simulink library "NCS_Library"  (R2019a)
settings: Solver=VariableStepAuto  StartTime=0.0  StopTime=10.0  RelTol=1e-3
values from neighbouring files (symbols this model uses):
  A = 10    [Parameter.m]
  band = 100000000    [Parameter.m]
  BER = 0    [Parameter.m]
  c = 5000000    [Parameter.m]
  c1 = 4.33    [Parameter.m]
  c2 = 3.16    [Parameter.m]
  CAN2EthernetDelay = 0.000    (= 0)    [Parameter.m]
  cR = 1.5*10^-3    (= 0.0015)    [Parameter.m]
  cw = (cwE * 2 + cwM * (nW_ges-2))/nW_ges    (= 0.1475)    [Parameter.m]
  cwE = 0.35    [Parameter.m]
  cwM = 0.08    [Parameter.m]
  Cycle_Controller = 0    [Parameter.m]
  CyclePLC = 24/1000    (= 0.024)    [Parameter.m]
  d = 800000    [Parameter.m]
  Dr = 0.92    [Parameter.m]
  Ethernet2CANDelay = 0.005    [Parameter.m]
  F_konst = 70892    [Parameter.m]
  FA = 100000    [Parameter.m]
  FB_WB_max = 10000    [Parameter.m]
  FBel_an = iG*nG*F_KZmax*nBan*R_mR/(Dr/2)    (= 28197.4297239)    [Parameter.m]
  FBel_frei = iG*nG*F_KZmax*nBfrei*R_mW/(Dr/2)    (= 29270.6882948)    [Parameter.m]
  Fmaxdyn = 300000    [Parameter.m]
  g = 9.81    [Parameter.m]
  i = 0    [Parameter.m]
  J = 1/2*mA*(Dr/2)^2    (= 158.7)    [Parameter.m]
  k1 = 0.095    [Parameter.m]
  k2 = 9.26/3.6    (= 2.57222222222)    [Parameter.m]
  k3 = 4.63/3.6    (= 1.28611111111)    [Parameter.m]
  mges = 58000    [Parameter.m]
  mu = [mu1 mu2]    [Parameter.m]
  muBel1 = 0.42    [Parameter.m]
  muBel2 = 0.36    [Parameter.m]
  n = 0.001    [Parameter.m]
  n_Mg = 4    [Parameter.m]
  n_WB = 4    [Parameter.m]
  nA = 4    [Parameter.m]
  nBan = 2    [Parameter.m]
  nBfrei = 3    [Parameter.m]
  nM = 4    [Parameter.m]
  nW_an = 4    [Parameter.m]
  P_max = 8200000    [Parameter.m]
  Q = 10    [Parameter.m]
  r_reib = 600    [Parameter.m]
  rho = 1.08    [Parameter.m]
  rhoL = 1.225    [Parameter.m]
  Size = 8    [Parameter.m]
  slip = [s1 s2]    [Parameter.m]
  tol = 0.05    [Parameter.m]
  v00 = 100/3.6    (= 27.7777777778)    [Parameter.m]
  v_grenz = 60/3.6    (= 16.6666666667)    [Parameter.m]
  v_opt = 75/3.6    (= 20.8333333333)    [Parameter.m]
  W_opt = 0.5    [Parameter.m]
  WB = 1    [Parameter.m]
  y_opt = sqrt(W_opt)/((1+sqrt(W_opt))^2+W_opt)    [Parameter.m]
undefined symbols (not defined in the file or in its folder): BUSCapacity, CableLength, controlGate, D_dyn, D_mg, EnableBurst, EnableToF, entity, Entity_out, Gate, Gate_4, Gate_5, Gate_ACK, Gate_copy, Gate_RX, getData, gettime, I_dyn, I_mg, m, magnitude, P_dyn, P_mg, ReadAttributes, readdata, ReadData, ReadSize, sigbuilder_block, Timeout, ToB, ToF, v0, v_d, v_soll
libraries: simulink x176, $bdroot x102
(part 10 of 12)

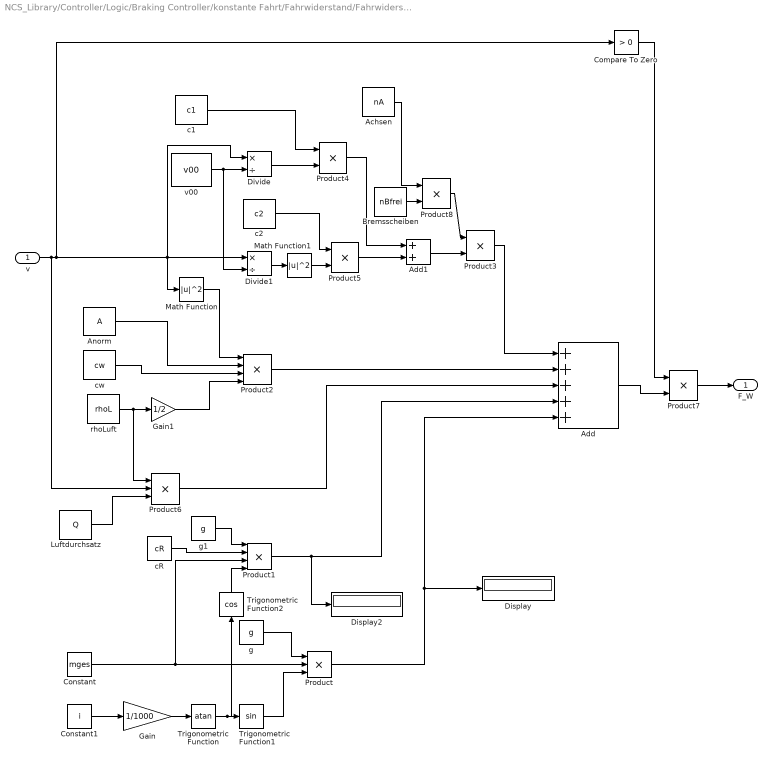
== system NCS_Library/Controller/Logic/Braking Controller/konstante Fahrt/Fahrwiderstand/Fahrwiderstand_freiWagen ==
  v : Inport
  Achsen : Constant  Value=nA
  Add : Sum  Inputs=+++++
  Add1 : Sum
  Anorm : Constant  Value=A
  Bremsscheiben : Constant  Value=nBfrei
  Compare To Zero : simulink/Logic and Bit Operations/Compare To Zero  relop=>  OutDataTypeStr=boolean
  Constant : Constant  Value=mges
  Constant1 : Constant  Value=i
  Display : Display
  Display2 : Display
  Divide : Product  Inputs=*/
  Divide1 : Product  Inputs=*/
  Gain : Gain  Gain=1/1000
  Gain1 : Gain  Gain=1/2
  Luftdurchsatz : Constant  Value=Q
  Math Function : Math  Operator=magnitude^2  SaturateOnIntegerOverflow=on
  Math Function1 : Math  Operator=magnitude^2  SaturateOnIntegerOverflow=on
  Product : Product  Inputs=3
  Product1 : Product  Inputs=4
  Product2 : Product  Inputs=4
  Product{3..5,7..8} (5 alike) : Product
  Product6 : Product  Inputs=3
  Trigonometric Function : Trigonometry  Operator=atan
  Trigonometric Function1 : Trigonometry
  Trigonometric Function2 : Trigonometry  Operator=cos
  c1 : Constant  Value=c1
  c2 : Constant  Value=c2
  cR : Constant  Value=cR
  cw : Constant  Value=cw
  g : Constant  Value=g
  g1 : Constant  Value=g
  rhoLuft : Constant  Value=rhoL
  v00 : Constant  Value=v00
  F_W : Outport
  wires:
  Trigonometric Function2/1 -> Product1/4
  Constant/1 -> Product1/3, Product/2
  cR/1 -> Product1/2
  g1/1 -> Product1/1
  Gain/1 -> Trigonometric Function/1
  Trigonometric Function/1 -> Trigonometric Function1/1, Trigonometric Function2/1
  Constant1/1 -> Gain/1
  Bremsscheiben/1 -> Product8/2
  Product8/1 -> Product3/1
  Compare To Zero/1 -> Product7/1
  Product7/1 -> F_W/1
  Math Function1/1 -> Product5/2
  Product6/1 -> Add/3
  Luftdurchsatz/1 -> Product6/3
  c2/1 -> Product5/1
  Math Function/1 -> Product2/1
  Divide1/1 -> Math Function1/1
  Product5/1 -> Add1/2
  Product4/1 -> Add1/1
  Divide/1 -> Product4/2
  v00/1 -> Divide/2, Divide1/2
  c1/1 -> Product4/1
  Add1/1 -> Product3/2
  Product3/1 -> Add/1
  Achsen/1 -> Product8/1
  Product2/1 -> Add/2
  Gain1/1 -> Product2/4
  cw/1 -> Product2/3
  Anorm/1 -> Product2/2
  v/1 -> Math Function/1, Divide/1, Divide1/1, Compare To Zero/1, Product6/2
  rhoLuft/1 -> Gain1/1, Product6/1
  Product1/1 -> Add/4, Display2/1
  Add/1 -> Product7/2
  Product/1 -> Add/5, Display/1
  Trigonometric Function1/1 -> Product/3
  g/1 -> Product/1

== system NCS_Library/Controller/Logic/Braking Controller/konstante Fahrt/WB Bremse pro Wagen/Subsystem ==
  v : Inport
  Add : Sum
  Add1 : Sum
  Berechnung W : Subsystem
  Compare To Zero : simulink/Logic and Bit Operations/Compare To Zero  relop=>=  OutDataTypeStr=boolean
  Constant : Constant
  Display : Display
  Divide : Product  Inputs=*/
  Math Function : Math  Operator=magnitude^2  SaturateOnIntegerOverflow=on
  Product : Product
  Scope : Scope
  Sqrt : Sqrt  SaturateOnIntegerOverflow=on
  y : Outport
  wires:
  Compare To Zero/1 -> Product/1
  Berechnung W/1(W) -> Product/2, Compare To Zero/1
  Add1/1 -> Divide/2
  Divide/1 -> Scope/1, y/1
  Math Function/1 -> Add1/1
  Add/1 -> Math Function/1
  Constant/1 -> Add/2
  Sqrt/1 -> Divide/1, Add/1
  Product/1 -> Sqrt/1, Add1/2, Display/1
  v/1 -> Berechnung W/1(v)

== system NCS_Library/Network/CAN/Logik/Fast_to_Slow/Measurement/Enabled Subsystem3 ==
  time_arrived : Inport
  time_sent : Inport  Port=2
  Enable : EnablePort
  Add : Sum  Inputs=+-
  delay : Outport
  wires:
  Add/1 -> delay/1
  time_sent/1 -> Add/2
  time_arrived/1 -> Add/1

== system NCS_Library/Network/CAN/Logik/Fast_to_Slow/Measurement/Simulink Function7 ==
  getData : TriggerPort  TriggerType=function-call  IsSimulinkFunction=on  FunctionName=getData  FunctionVisibility=scoped  VariantControl=Variant
  u1 : ArgIn  DisableCoverage=on  ArgumentName=time
  time : Outport  InitialOutput=-1
  wires:
  u1/1 -> time/1

== system NCS_Library/Network/CAN/Logik/Fast_to_Slow/Slow Takt/Simulink Function3 ==
  Gate_5 : TriggerPort  TriggerType=function-call  IsSimulinkFunction=on  FunctionName=Gate_5  FunctionVisibility=scoped  VariantControl=Variant
  Message Send : MessageSend  OutputPortMessageModes=m
      settings: InputPortMap=u1
  u : ArgIn  DisableCoverage=on  ArgumentName=u
  ctrl : Outport  InitialOutput=0
  wires:
  Message Send/1 -> ctrl/1
  u/1 -> Message Send/1

== system NCS_Library/Network/CAN/Logik/Fast_to_Slow/Wait Takt/Simulink Function3 ==
  Gate_4 : TriggerPort  TriggerType=function-call  IsSimulinkFunction=on  FunctionName=Gate_4  FunctionVisibility=scoped  VariantControl=Variant
  Message Send : MessageSend  OutputPortMessageModes=m
      settings: InputPortMap=u1
  u : ArgIn  DisableCoverage=on  ArgumentName=u
  ctrl : Outport  InitialOutput=0
  wires:
  u/1 -> Message Send/1
  Message Send/1 -> ctrl/1

== system NCS_Library/Network/CAN/Logik/Slow_to_Fast/Copy Takt/Simulink Function3 ==
  Gate_copy : TriggerPort  TriggerType=function-call  IsSimulinkFunction=on  FunctionName=Gate_copy  FunctionVisibility=scoped  VariantControl=Variant
  Message Send : MessageSend  OutputPortMessageModes=m
      settings: InputPortMap=u1
  u : ArgIn  DisableCoverage=on  ArgumentName=u
  ctrl : Outport  InitialOutput=0
  wires:
  u/1 -> Message Send/1
  Message Send/1 -> ctrl/1

== system NCS_Library/Network/CAN/Logik/Slow_to_Fast/Fast Takt/Simulink Function3 ==
  Gate : TriggerPort  TriggerType=function-call  IsSimulinkFunction=on  FunctionName=Gate  FunctionVisibility=scoped  VariantControl=Variant
  Message Send : MessageSend  OutputPortMessageModes=m
      settings: InputPortMap=u1
  u : ArgIn  DisableCoverage=on  ArgumentName=u
  ctrl : Outport  InitialOutput=0
  wires:
  u/1 -> Message Send/1
  Message Send/1 -> ctrl/1

== system NCS_Library/Network/CAN/Logik/Slow_to_Fast/Logic Takt/Simulink Function3 ==
  Gate : TriggerPort  TriggerType=function-call  IsSimulinkFunction=on  FunctionName=Gate  FunctionVisibility=scoped  VariantControl=Variant
  Message Send : MessageSend  OutputPortMessageModes=m
      settings: InputPortMap=u1
  u : ArgIn  DisableCoverage=on  ArgumentName=u
  ctrl : Outport  InitialOutput=0
  wires:
  Message Send/1 -> ctrl/1
  u/1 -> Message Send/1

== system NCS_Library/Network/CAN/Logik/Slow_to_Fast/Measurement/Enabled Subsystem ==
  time_arrived : Inport
  time : Inport  Port=2
  Enable : EnablePort
  Add : Sum  Inputs=+-
  delay : Outport
  wires:
  time_arrived/1 -> Add/1
  time/1 -> Add/2
  Add/1 -> delay/1

== system NCS_Library/Network/CAN/Logik/Slow_to_Fast/Measurement/Fast Takt ==
  In : Inport
  Entity Takt : EntityGenerator  OutputPortMessageModes=m  TimeSource=Signal port  Period=7  AttributeName=entity  EntityTypeName=gate  EntityPriority=10  DataInitialValue=1
      settings: InputPortMap=u1
  Entity Terminator13 : EntityTerminator  InputPortMessageModes=m
  Gate : EntityGate  InputPortMessageModes=m,m  OutputPortMessageModes=m
  Offset [s] : Constant  Value=Offset
  Server : EntityServer  InputPortMessageModes=m  OutputPortMessageModes=m  Capacity=1  ServiceTimeValue=0  EntryAction=Gate(0);
  Server Offset : EntityServer  InputPortMessageModes=n,m  OutputPortMessageModes=m  Capacity=inf  ServiceTimeSource=Signal port  ServiceTimeValue=5
      settings: InputPortMap=u0,u2
  Server Takt : EntityServer  InputPortMessageModes=m  OutputPortMessageModes=m  Capacity=1  ServiceTimeValue=0.001  ServiceTimeAttributeName=CommDelay  EntryAction=Gate(1);  ExitAction=Gate(0);  SortingAttributeName=ID
  Simulink Function3 : Subsystem  TreatAsAtomicUnit=on
  Takt_fast [s] : Constant  Value=Takt_fast
  Out : Outport
  wires:
  Offset [s]/1 -> Server Offset/1
  Takt_fast [s]/1 -> Entity Takt/1
  Server Takt/1 -> Entity Terminator13/1
  Server Offset/1 -> Server Takt/1
  Entity Takt/1 -> Server Offset/2
  Simulink Function3/1(ctrl) -> Gate/1
  In/1 -> Gate/2
  Gate/1 -> Server/1
  Server/1 -> Out/1

== system NCS_Library/Network/CAN/Logik/Slow_to_Fast/Measurement/Simulink Function6 ==
  getData : TriggerPort  TriggerType=function-call  IsSimulinkFunction=on  FunctionName=getData  FunctionVisibility=scoped  VariantControl=Variant
  u : ArgIn  DisableCoverage=on  ArgumentName=time
  time : Outport  InitialOutput=-1
  wires:
  u/1 -> time/1

== system NCS_Library/Network/ETB/Burst Device/Protocl Stack/TRDP PD/Enabled Subsystem1 ==
  msgType : Inport
  ReplyAddress : Inport  Port=2
  Enable : EnablePort
  MATLAB Function : MATLAB Function  TreatAsAtomicUnit=on
  msgTypeReply : Outport  OutputWhenDisabled=reset  InitialOutput=0
  DestinationReply : Outport  Port=2
  wires:
  MATLAB Function/1(msgTypeReply) -> msgTypeReply/1
  ReplyAddress/1 -> DestinationReply/1
  msgType/1 -> MATLAB Function/1(msgType)

== system NCS_Library/Network/ETB/Burst Device/Protocl Stack/TRDP PD/Simulink Function ==
  msgType : Inport
  Destination : Inport  Port=2
  Source : Inport  Port=3
  UDP : Inport  Port=4
  ReplyAddress : Inport  Port=5
  f : TriggerPort  TriggerType=function-call  IsSimulinkFunction=on  FunctionName=SetAttributes  FunctionVisibility=scoped  VariantControl=(inherit)
  Constant : Constant  OutDataTypeStr=uint8
  Display : Display
  MATLAB Function : MATLAB Function  TreatAsAtomicUnit=on
  SSC : ArgIn  DisableCoverage=on  OutDataTypeStr=uint32  ArgumentName=SSC
  SSC1 : ArgIn  DisableCoverage=on  Port=2  PortDimensions=[3 20]  ArgumentName=Data
  y : ArgOut  DisableCoverage=on  OutDataTypeStr=uint32  ArgumentName=SEQ
  y1 : ArgOut  DisableCoverage=on  Port=2  OutDataTypeStr=uint8  ArgumentName=msgType
  y2 : ArgOut  DisableCoverage=on  Port=3  OutDataTypeStr=uint16  PortDimensions=[1 4]  ArgumentName=Destination
  y3 : ArgOut  DisableCoverage=on  Port=4  OutDataTypeStr=uint16  PortDimensions=[1 4]  ArgumentName=Source
  y5 : ArgOut  DisableCoverage=on  Port=5  OutDataTypeStr=uint8  ArgumentName=CheckBit
  y4 : ArgOut  DisableCoverage=on  Port=6  PortDimensions=[3 20]  ArgumentName=Data
  y6 : ArgOut  DisableCoverage=on  Port=7  OutDataTypeStr=uint16  ArgumentName=UDP
  y7 : ArgOut  DisableCoverage=on  Port=8  OutDataTypeStr=uint16  PortDimensions=[ 1 4 ]  ArgumentName=ReplyAddress
  wires:
  ReplyAddress/1 -> y7/1
  UDP/1 -> y6/1
  MATLAB Function/1(Data_edited) -> y4/1
  SSC1/1 -> MATLAB Function/1(Data)
  Constant/1 -> y5/1
  SSC/1 -> y/1
  Source/1 -> y3/1
  Destination/1 -> y2/1, Display/1
  msgType/1 -> y1/1, MATLAB Function/2(msgType)

== system NCS_Library/Network/ETB/Burst Device/Protocl Stack/TRDP PD/Simulink Function1 ==
  ReadData : TriggerPort  TriggerType=function-call  IsSimulinkFunction=on  FunctionName=ReadData  FunctionVisibility=scoped  VariantControl=(inherit)
  MATLAB Function : MATLAB Function  TreatAsAtomicUnit=on
  MATLAB Function2 : MATLAB Function  TreatAsAtomicUnit=on
  SourceAddress : ArgIn  DisableCoverage=on  OutDataTypeStr=uint8  ArgumentName=msgType
  SourceAddress1 : ArgIn  DisableCoverage=on  Port=2  OutDataTypeStr=uint16  PortDimensions=[1 4]  ArgumentName=Reply
  SourceAddress2 : ArgIn  DisableCoverage=on  Port=3  OutDataTypeStr=uint16  PortDimensions=[1 4]  ArgumentName=Source
  msgType : Outport  OutDataTypeStr=uint8  OutputWhenDisabled=reset  InitialOutput=0
  ReplyAddress : Outport  Port=2  OutDataTypeStr=uint16
  wires:
  MATLAB Function2/1(DestinationPull) -> ReplyAddress/1
  SourceAddress/1 -> MATLAB Function2/1(msgType), msgType/1
  MATLAB Function/1(Address) -> MATLAB Function2/2(ReplyAddress)
  SourceAddress2/1 -> MATLAB Function/2(Source)
  SourceAddress1/1 -> MATLAB Function/1(Reply)

== system NCS_Library/Network/ETB/OSI Layers/MAC Controller/CSMA//CD/Discrete Event Subsystem (Carrier Sensing)1 ==
  l_status : Inport
  Compare To Zero1 : simulink/Logic and Bit Operations/Compare To Zero  relop=>  OutDataTypeStr=boolean
  Constant1 : Constant
  Sum1 : Sum  Inputs=|+-
  l_ready : Outport  InitialOutput=1
  wires:
  Compare To Zero1/1 -> l_ready/1
  Sum1/1 -> Compare To Zero1/1
  l_status/1 -> Sum1/2
  Constant1/1 -> Sum1/1

== system NCS_Library/Network/ETB/OSI Layers/SDTv2/Safety Measures/Latency Monitoring ==
  Timestamp : Inport
  T_rx_safe : Inport  Port=2
  Enable : EnablePort
  Add1 : Sum  Inputs=+--+
  Clock : Clock
  Compare To Zero1 : simulink/Logic and Bit Operations/Compare To Zero  relop=>=  OutDataTypeStr=uint8
  Constant : Constant  Value=1e-8
  Contration Phase : Outport  InitialOutput=0
  wires:
  Add1/1 -> Compare To Zero1/1
  Compare To Zero1/1 -> Contration Phase/1
  T_rx_safe/1 -> Add1/3
  Timestamp/1 -> Add1/2
  Clock/1 -> Add1/1
  Constant/1 -> Add1/4  "compensate numerical drift"

== system NCS_Library/Network/ETB/OSI Layers/SDTv2/Safety Measures/Sink-Time Supervision ==
  T_rx_safe : Inport
  SSC : Inport  Port=2
  Add : Sum
  Add2 : Sum  Inputs=-+-+
  Clock1 : Clock
  Compare To Zero : simulink/Logic and Bit Operations/Compare To Zero  relop===  OutDataTypeStr=boolean
  Compare To Zero2 : simulink/Logic and Bit Operations/Compare To Zero  relop=>=  OutDataTypeStr=uint8
  Constant1 : Constant  Value=1e-10
  Detect Change : simulink/Logic and Bit Operations/Detect Change  vinit=0  OutDataTypeStr=uint8
  Save last time : Subsystem
  LSC : Outport  InitialOutput=0
  wires:
  Detect Change/1 -> Add/2
  Compare To Zero/1 -> Add/1
  SSC/1 -> Detect Change/1, Compare To Zero/1
  Add2/1 -> Compare To Zero2/1
  Constant1/1 -> Add2/4  "Compensate numeric drift"
  T_rx_safe/1 -> Add2/3
  Compare To Zero2/1 -> LSC/1  "loss of safe communication"
  Add/1 -> Save last time/Enable
  Save last time/1(Out1) -> Add2/1
  Clock1/1 -> Save last time/1(Time), Add2/2

== system NCS_Library/Network/ETB/OSI Layers/SDTv2/Safety Measures/Subsystem ==
  note: Ensure computing delay for every fresh VDP except inital
  In1 : Inport
  Add : Sum  Inputs=++-
  Compare To Zero : simulink/Logic and Bit Operations/Compare To Zero  relop=>  OutDataTypeStr=boolean
  Compare To Zero1 : simulink/Logic and Bit Operations/Compare To Zero  relop=>  OutDataTypeStr=boolean
  Constant : Constant
  Delay : Delay  DelayLength=1
  Detect Change : simulink/Logic and Bit Operations/Detect Change  vinit=0  OutDataTypeStr=boolean
  Out1 : Outport
  wires:
  Add/1 -> Compare To Zero1/1
  In1/1 -> Compare To Zero/1, Detect Change/1
  Detect Change/1 -> Add/2  "Fresh VDP"
  Constant/1 -> Add/3
  Compare To Zero1/1 -> Out1/1
  Delay/1 -> Add/1  "Open Connection"
  Compare To Zero/1 -> Delay/1

== system NCS_Library/Network/ETB/OSI Layers/SDTv2/Subsystem/Save last release time ==
  Time : Inport
  Enable : EnablePort
  Add : Sum
  Constant : Constant  OutDataTypeStr=uint32
  Data Type Conversion : DataTypeConversion  OutDataTypeStr=double
  Display : Display
  Out1 : Outport  InitialOutput=0
  wires:
  Time/1 -> Add/1
  Add/1 -> Data Type Conversion/1
  Constant/1 -> Add/2
  Data Type Conversion/1 -> Display/1, Out1/1

== system NCS_Library/Network/ETB/OSI Layers/TRDP PD/Detect Event/Enabled Subsystem ==
  In1 : Inport
  Enable : EnablePort
  Out1 : Outport  OutputWhenDisabled=reset  InitialOutput=0
  wires:
  In1/1 -> Out1/1

== system NCS_Library/Network/ETB/OSI Layers/TRDP PD/Subsystem/Save last release time ==
  n : Inport
  Enable : EnablePort
  Add : Sum
  Constant : Constant  OutDataTypeStr=uint32
  Data Type Conversion : DataTypeConversion  OutDataTypeStr=double
  Display : Display
  n_new : Outport  InitialOutput=0
  wires:
  n/1 -> Add/1
  Add/1 -> Data Type Conversion/1
  Constant/1 -> Add/2
  Data Type Conversion/1 -> Display/1, n_new/1

== system NCS_Library/Network/ETB/Subsystem2/Routing Layer/Logic 1/Simulink Function1 ==
  Parameter : Inport
  RT : Inport  Port=2
  Routing : TriggerPort  TriggerType=function-call  IsSimulinkFunction=on  FunctionName=Routing  FunctionVisibility=scoped  VariantControl=(inherit)
  Add : Sum  Inputs=+-
  Bus Selector1 : BusSelector  OutputSignals=SubnetID1,SubnetID2,SubnetID3
  Compare To Zero : simulink/Logic and Bit Operations/Compare To Zero  relop===  OutDataTypeStr=uint8
  Constant : Constant  Value=RouterID  OutDataTypeStr=uint16
  Constant1 : Constant  OutDataTypeStr=uint8
  Constant2 : Constant  Value=RouterID  OutDataTypeStr=uint16
  Data Type Conversion : DataTypeConversion  OutDataTypeStr=uint8
  Display : Display
  MATLAB Function : MATLAB Function  TreatAsAtomicUnit=on
  Switch : Switch  Criteria=u2 > Threshold  OutDataTypeStr=uint8
  Switch1 : Switch  Criteria=u2 > Threshold
  Destination : ArgIn  DisableCoverage=on  OutDataTypeStr=uint16  PortDimensions=[1 4]  ArgumentName=Destination
  InID : ArgIn  DisableCoverage=on  Port=2  OutDataTypeStr=uint8  ArgumentName=InID
  Route : ArgOut  DisableCoverage=on  OutDataTypeStr=uint8  ArgumentName=Route
  MACSource : ArgOut  DisableCoverage=on  Port=2  OutDataTypeStr=uint16  ArgumentName=MACSource
  MACDestination : ArgOut  DisableCoverage=on  Port=3  OutDataTypeStr=uint16  ArgumentName=MACDestination
  OutID : ArgOut  DisableCoverage=on  Port=4  OutDataTypeStr=uint8  ArgumentName=OutID
  wires:
  MATLAB Function/2(Route) -> Data Type Conversion/1
  RT/1 -> MATLAB Function/5(RT)
  Destination/1 -> MATLAB Function/4(Destination)
  Data Type Conversion/1 -> Switch1/3, Display/1
  Bus Selector1/1 -> MATLAB Function/1(S1)  "<SubnetID1>"
  Bus Selector1/2 -> MATLAB Function/2(S2)  "<SubnetID2>"
  Bus Selector1/3 -> MATLAB Function/3(S3)  "<SubnetID3>"
  Parameter/1 -> Bus Selector1/1
  Constant/1 -> MACSource/1
  MATLAB Function/1(MACDestination) -> MACDestination/1
  Compare To Zero/1 -> Switch1/2
  Add/1 -> Compare To Zero/1
  InID/1 -> Switch/2, Switch/1, Add/2
  Switch/1 -> OutID/1
  Constant2/1 -> Switch/3, Add/1
  Switch1/1 -> Route/1
  Constant1/1 -> Switch1/1

== system NCS_Library/Network/ETB/Subsystem2/Routing Layer/Logic 1/Subsystem ==
  In1 : Inport
  Constant : Constant
  Message Send : MessageSend  OutputPortMessageModes=m  ShowEnablePort=on
      settings: InputPortMap=e0,u1
  Out1 : Outport
  wires:
  In1/1 -> Message Send/1
  Message Send/1 -> Out1/1
  Constant/1 -> Message Send/2

== system NCS_Library/Network/ETB/Subsystem2/Routing Layer/Logic 2/Simulink Function1 ==
  Parameter : Inport
  RT : Inport  Port=2
  Routing : TriggerPort  TriggerType=function-call  IsSimulinkFunction=on  FunctionName=Routing  FunctionVisibility=scoped  VariantControl=(inherit)
  Add : Sum  Inputs=+-
  Bus Selector1 : BusSelector  OutputSignals=SubnetID1,SubnetID2,SubnetID3
  Compare To Zero : simulink/Logic and Bit Operations/Compare To Zero  relop===  OutDataTypeStr=uint8
  Constant : Constant  Value=RouterID  OutDataTypeStr=uint16
  Constant1 : Constant  Value=2  OutDataTypeStr=uint8
  Constant2 : Constant  Value=RouterID  OutDataTypeStr=uint16
  Data Type Conversion : DataTypeConversion  OutDataTypeStr=uint8
  Display : Display
  MATLAB Function : MATLAB Function  TreatAsAtomicUnit=on
  Switch : Switch  Criteria=u2 > Threshold  OutDataTypeStr=uint8
  Switch1 : Switch  Criteria=u2 > Threshold
  Destination : ArgIn  DisableCoverage=on  OutDataTypeStr=uint16  PortDimensions=[1 4]  ArgumentName=Destination
  InID : ArgIn  DisableCoverage=on  Port=2  OutDataTypeStr=uint8  ArgumentName=InID
  Route : ArgOut  DisableCoverage=on  OutDataTypeStr=uint8  ArgumentName=Route
  MACSource : ArgOut  DisableCoverage=on  Port=2  OutDataTypeStr=uint16  ArgumentName=MACSource
  MACDestination : ArgOut  DisableCoverage=on  Port=3  OutDataTypeStr=uint16  ArgumentName=MACDestination
  OutID : ArgOut  DisableCoverage=on  Port=4  OutDataTypeStr=uint8  ArgumentName=OutID
  wires:
  MATLAB Function/2(Route) -> Data Type Conversion/1
  RT/1 -> MATLAB Function/5(RT)
  Destination/1 -> MATLAB Function/4(Destination)
  Data Type Conversion/1 -> Switch1/3, Display/1
  Bus Selector1/1 -> MATLAB Function/1(S1)  "<SubnetID1>"
  Bus Selector1/2 -> MATLAB Function/2(S2)  "<SubnetID2>"
  Bus Selector1/3 -> MATLAB Function/3(S3)  "<SubnetID3>"
  Parameter/1 -> Bus Selector1/1
  Constant/1 -> MACSource/1
  MATLAB Function/1(MACDestination) -> MACDestination/1
  Compare To Zero/1 -> Switch1/2
  Add/1 -> Compare To Zero/1
  InID/1 -> Switch/2, Switch/1, Add/2
  Switch/1 -> OutID/1
  Constant2/1 -> Switch/3, Add/1
  Switch1/1 -> Route/1
  Constant1/1 -> Switch1/1

== system NCS_Library/Network/ETB/Subsystem2/Routing Layer/Logic 2/Subsystem ==
  In1 : Inport
  Constant : Constant
  Message Send : MessageSend  OutputPortMessageModes=m  ShowEnablePort=on
      settings: InputPortMap=e0,u1
  Out1 : Outport
  wires:
  In1/1 -> Message Send/1
  Message Send/1 -> Out1/1
  Constant/1 -> Message Send/2

== system NCS_Library/Network/ETB/Subsystem2/Routing Layer/Logic 3/Simulink Function ==
  In1 : Inport
  Flooding : TriggerPort  TriggerType=function-call  IsSimulinkFunction=on  FunctionName=Flooding  FunctionVisibility=scoped  VariantControl=(inherit)
  Add : Sum  Inputs=+-
  Add1 : Sum
  Bus Selector : BusSelector  OutputSignals=RouterID
  Compare To Zero : simulink/Logic and Bit Operations/Compare To Zero  relop===  OutDataTypeStr=uint8
  Constant : Constant  OutDataTypeStr=uint8
  Constant1 : Constant  Value=RouterID  OutDataTypeStr=uint16
  Switch : Switch  Criteria=u2 > Threshold
  u : ArgIn  DisableCoverage=on  OutDataTypeStr=uint8  ArgumentName=InID
  y : ArgOut  DisableCoverage=on  OutDataTypeStr=uint8  ArgumentName=OutID
  y1 : ArgOut  DisableCoverage=on  Port=2  OutDataTypeStr=uint8  ArgumentName=Route
  MACSource : ArgOut  DisableCoverage=on  Port=3  OutDataTypeStr=uint16  ArgumentName=MACSource
  wires:
  u/1 -> Add/2, Switch/1, Switch/2
  Switch/1 -> y/1
  Bus Selector/1 -> Switch/3, Add/1  "<RouterID>"
  In1/1 -> Bus Selector/1
  Add/1 -> Compare To Zero/1
  Compare To Zero/1 -> Add1/2
  Constant/1 -> Add1/1
  Add1/1 -> y1/1
  Constant1/1 -> MACSource/1

== system NCS_Library/Network/ETB/Subsystem2/Routing Layer/Logic 3/Simulink Function1 ==
  Parameter : Inport
  RT : Inport  Port=2
  Routing : TriggerPort  TriggerType=function-call  IsSimulinkFunction=on  FunctionName=Routing  FunctionVisibility=scoped  VariantControl=(inherit)
  Add : Sum  Inputs=+-
  Bus Selector1 : BusSelector  OutputSignals=SubnetID1,SubnetID2,SubnetID3
  Compare To Zero : simulink/Logic and Bit Operations/Compare To Zero  relop===  OutDataTypeStr=uint8
  Constant : Constant  Value=RouterID  OutDataTypeStr=uint16
  Constant1 : Constant  Value=3  OutDataTypeStr=uint8
  Constant2 : Constant  Value=RouterID  OutDataTypeStr=uint16
  Data Type Conversion : DataTypeConversion  OutDataTypeStr=uint8
  Display : Display
  MATLAB Function : MATLAB Function  TreatAsAtomicUnit=on
  Switch : Switch  Criteria=u2 > Threshold  OutDataTypeStr=uint8
  Switch1 : Switch  Criteria=u2 > Threshold
  Destination : ArgIn  DisableCoverage=on  OutDataTypeStr=uint16  PortDimensions=[1 4]  ArgumentName=Destination
  InID : ArgIn  DisableCoverage=on  Port=2  OutDataTypeStr=uint8  ArgumentName=InID
  Route : ArgOut  DisableCoverage=on  OutDataTypeStr=uint8  ArgumentName=Route
  MACSource : ArgOut  DisableCoverage=on  Port=2  OutDataTypeStr=uint16  ArgumentName=MACSource
  MACDestination : ArgOut  DisableCoverage=on  Port=3  OutDataTypeStr=uint16  ArgumentName=MACDestination
  OutID : ArgOut  DisableCoverage=on  Port=4  OutDataTypeStr=uint8  ArgumentName=OutID
  wires:
  MATLAB Function/2(Route) -> Data Type Conversion/1
  RT/1 -> MATLAB Function/5(RT)
  Destination/1 -> MATLAB Function/4(Destination)
  Data Type Conversion/1 -> Switch1/3, Display/1
  Bus Selector1/1 -> MATLAB Function/1(S1)  "<SubnetID1>"
  Bus Selector1/2 -> MATLAB Function/2(S2)  "<SubnetID2>"
  Bus Selector1/3 -> MATLAB Function/3(S3)  "<SubnetID3>"
  Parameter/1 -> Bus Selector1/1
  Constant/1 -> MACSource/1
  MATLAB Function/1(MACDestination) -> MACDestination/1
  Compare To Zero/1 -> Switch1/2
  Add/1 -> Compare To Zero/1
  InID/1 -> Switch/2, Switch/1, Add/2
  Switch/1 -> OutID/1
  Constant2/1 -> Switch/3, Add/1
  Switch1/1 -> Route/1
  Constant1/1 -> Switch1/1

== system NCS_Library/Network/ETB/Subsystem2/Routing Layer/Logic 3/Subsystem ==
  In1 : Inport
  Constant : Constant
  Message Send : MessageSend  OutputPortMessageModes=m  ShowEnablePort=on
      settings: InputPortMap=e0,u1
  Out1 : Outport
  wires:
  In1/1 -> Message Send/1
  Message Send/1 -> Out1/1
  Constant/1 -> Message Send/2

== system NCS_Library/Network/ETB/Subsystem2/Routing Table/Get Routing Table/Compute Routing Table ==
  ID : Inport
  RM : Inport  Port=2
  Enable : EnablePort
  Constant : Constant
  Data Type Conversion : DataTypeConversion  OutDataTypeStr=double
  Data Type Conversion1 : DataTypeConversion  OutDataTypeStr=double
  Data Type Conversion2 : DataTypeConversion  OutDataTypeStr=uint16
  MATLAB Function : MATLAB Function  TreatAsAtomicUnit=on
  FIN_Init : Outport  OutputWhenDisabled=reset  InitialOutput=0
  RT : Outport  Port=2  OutDataTypeStr=uint16
  wires:
  Constant/1 -> FIN_Init/1
  Data Type Conversion2/1 -> RT/1
  Data Type Conversion1/1 -> MATLAB Function/2(RM)
  Data Type Conversion/1 -> MATLAB Function/1(ID)
  MATLAB Function/1(RT) -> Data Type Conversion2/1
  RM/1 -> Data Type Conversion1/1
  ID/1 -> Data Type Conversion/1

== system NCS_Library/Network/ETB/Subsystem2/Routing Table/Get Routing Table/Compute routing matrix RM ==
  RM_in : Inport
  Enable : EnablePort
  Display : Display
  Display1 : Display
  MATLAB Function : MATLAB Function  TreatAsAtomicUnit=on
  Memory : Memory
  Memory1 : Memory  InitialCondition=1  InheritSampleTime=on
  FIN_RM : Outport  OutputWhenDisabled=reset  InitialOutput=0
  RM_global : Outport  Port=2
  wires:
  RM_in/1 -> MATLAB Function/2(RM_in)
  MATLAB Function/2(FIN) -> FIN_RM/1
  MATLAB Function/1(state_out) -> Memory1/1
  Memory1/1 -> Display1/1, MATLAB Function/1(state)
  MATLAB Function/3(RM_global) -> Memory/1
  Memory/1 -> MATLAB Function/3(RM_old), RM_global/1, Display/1

== system NCS_Library/Network/ETB/Subsystem2/Routing Table/Get Routing Table/Simulink Function1 ==
  In1 : Inport
  s1 : Inport  Port=2
  In8 : Inport  Port=3
  In9 : Inport  Port=4
  In10 : Inport  Port=5
  In11 : Inport  Port=6
  Failed : Inport  Port=7
  writedata : TriggerPort  TriggerType=function-call  IsSimulinkFunction=on  FunctionName=writedata  FunctionVisibility=scoped  VariantControl=(inherit)
  Compute local routing matrix : MATLAB Function  TreatAsAtomicUnit=on
  Display : Display
  Logical Operator : Logic  Operator=NOT  Inputs=1  AllPortsSameDT=off  OutDataTypeStr=boolean
  Multiply : Product
  Mux : Mux  Inputs=5
  ID : ArgOut  DisableCoverage=on  PortDimensions=[10 2]  ArgumentName=R_local
  wires:
  In10/1 -> Mux/4
  In9/1 -> Mux/3
  In8/1 -> Mux/2
  s1/1 -> Mux/1
  In1/1 -> Compute local routing matrix/1(ID)
  Mux/1 -> Compute local routing matrix/2(s)
  In11/1 -> Mux/5
  Compute local routing matrix/1(R_local) -> Multiply/1
  Multiply/1 -> ID/1, Display/1
  Failed/1 -> Logical Operator/1
  Logical Operator/1 -> Multiply/2

== system NCS_Library/Network/ETB/Subsystem2/Routing Table/Get Routing Table/Simulink Function2 ==
  readdata : TriggerPort  TriggerType=function-call  IsSimulinkFunction=on  FunctionName=readdata  FunctionVisibility=scoped  VariantControl=(inherit)
  Compare To Zero : simulink/Logic and Bit Operations/Compare To Zero  relop===  OutDataTypeStr=boolean
  Display : Display
  MATLAB Function1 : MATLAB Function  TreatAsAtomicUnit=on
  ID : ArgIn  DisableCoverage=on  PortDimensions=[10 2]  ArgumentName=R_local
  RM_in : Outport
  Refresh : Outport  Port=2  InitialOutput=0
  wires:
  Compare To Zero/1 -> Refresh/1
  MATLAB Function1/1(Header) -> Compare To Zero/1
  ID/1 -> RM_in/1, MATLAB Function1/1(R_local), Display/1

== system NCS_Library/Network/Gateway/Gateway1/CAN Interface/CAN Interface/Re-Transmission Control ==
  IN : Inport
  ReTX : Inport  Port=2
  Reset : Inport  Port=3
  Discard Saved Message upon Success : EntityGate  InputPortMessageModes=m,m  OutputPortMessageModes=m  OperatingMode=Release gate
  Entity Sink : EntityTerminator  InputPortMessageModes=m  NumberEntitiesArrived=on
      settings: OutputPortMap=o0
  Re-Transmission Decision : EntityOutputSwitch  InputPortMessageModes=m  OutputPortMessageModes=m,m  SwitchAttributeName=Attribute1
  Re-transmit Saved Message upon Failure : EntityGate  InputPortMessageModes=m,m  OutputPortMessageModes=m  OperatingMode=Release gate
  OUT : Outport
  #TX : Outport  Port=2
  wires:
  IN/1 -> Re-Transmission Decision/1
  Re-Transmission Decision/1 -> Re-transmit Saved Message upon Failure/2
  Re-transmit Saved Message upon Failure/1 -> OUT/1
  Re-Transmission Decision/2 -> Discard Saved Message upon Success/2
  Discard Saved Message upon Success/1 -> Entity Sink/1
  Entity Sink/1 -> #TX/1
  ReTX/1 -> Re-transmit Saved Message upon Failure/1
  Reset/1 -> Discard Saved Message upon Success/1

== system NCS_Library/Network/Gateway/Gateway1/CAN Interface/CAN Interface/Reception Control/Compute ==
  rx_id : Inport  OutDataTypeStr=double  PortDimensions=1
  loss : Inport  Port=2  OutDataTypeStr=double  PortDimensions=1
  rx_rtr : Inport  Port=3  OutDataTypeStr=double  PortDimensions=1
  rx_data : Inport  Port=4  OutDataTypeStr=double  PortDimensions=1
  tx_id : Inport  Port=5  OutDataTypeStr=double  PortDimensions=1
  tx_rtr : Inport  Port=6  OutDataTypeStr=double  PortDimensions=1
  tx_data : Inport  Port=7  OutDataTypeStr=double  PortDimensions=1
  f : TriggerPort  TriggerType=function-call  VariantControl=Variant
      settings: CopyFcn=Stateflow.SLINSF.SimulinkMan.removeBlockPreDeleteFcn  PreDeleteFcn=Stateflow.SLINSF.SimulinkMan.unsafePredeleteFcn
  Lookup Table : Lookup  InputValues=IDRange  Table=2*ones(1,length(IDRange))-IDSubscription  LUTDesignUseExistingBP=off  LUTDesignAbsError=NaN
  MATLAB Function : MATLAB Function  TreatAsAtomicUnit=on
  Sum : Sum  Inputs=|++
  Status : Outport
  Ack : Outport  Port=2
  wires:
  MATLAB Function/1(ACK) -> Ack/1
  Sum/1 -> Status/1
  tx_rtr/1 -> MATLAB Function/5(RTR1)
  tx_data/1 -> MATLAB Function/6(Data1)
  rx_data/1 -> MATLAB Function/3(Data0)
  loss/1 -> MATLAB Function/7(Loss), Sum/2
  Lookup Table/1 -> Sum/1
  rx_id/1 -> Lookup Table/1, MATLAB Function/1(ID0)
  rx_rtr/1 -> MATLAB Function/2(RTR0)
  tx_id/1 -> MATLAB Function/4(ID1)

== system NCS_Library/Network/Gateway/Gateway1/CAN Interface/CAN Interface/Signal To CAN Message ==
  Data : Inport
  Entity Generator : EntityGenerator  OutputPortMessageModes=m  Period=T_Tx_CAN  GenerateEntityAtSimulationStart=off  GenerateAction=[entity.ID,entity.RTR,entity.Size,entity.f_St,entity.CommDelay,entity.Time, entity.SensorType] = initMessage();  AttributeName=ID|RTR|Size|Data|CommDelay|RndLoss  AttributeInitialValue=1|1|1|1|1|0  EntityType=Bus object  EntityTypeName=CAN_Message  EntityPriority=MsgID
  Set the Attributes of Messages : Subsystem  TreatAsAtomicUnit=on
  MsgOut : Outport
  wires:
  Entity Generator/1 -> MsgOut/1
  Data/1 -> Set the Attributes of Messages/1(InData)

== system NCS_Library/Network/Gateway/Gateway1/CAN Interface/CAN Interface/Simulink Function ==
  controlGate : TriggerPort  TriggerType=function-call  IsSimulinkFunction=on  FunctionName=controlGate  FunctionVisibility=scoped  VariantControl=Variant
  Message Send : MessageSend  OutputPortMessageModes=m
      settings: InputPortMap=u1
  u : ArgIn  DisableCoverage=on  ArgumentName=u
  ctrl : Outport
  wires:
  Message Send/1 -> ctrl/1
  u/1 -> Message Send/1

== system NCS_Library/Network/Gateway/Gateway1/CAN Interface/Entry Control/Enabled Subsystem ==
  Enable : EnablePort  StatesWhenEnabling=reset
  Constant : Constant
  Message Send3 : MessageSend  OutputPortMessageModes=m
      settings: InputPortMap=u1
  Out1 : Outport  OutputWhenDisabled=reset  InitialOutput=1
  wires:
  Constant/1 -> Message Send3/1
  Message Send3/1 -> Out1/1

== system NCS_Library/Network/Gateway/Gateway1/CAN Interface/Gate Control/Save last release time1 ==
  Time : Inport
  Enable : EnablePort
  Add : Sum
  Constant : Constant  OutDataTypeStr=uint32
  Data Type Conversion : DataTypeConversion  OutDataTypeStr=double
  Display : Display
  Out1 : Outport  InitialOutput=0
  wires:
  Data Type Conversion/1 -> Out1/1, Display/1
  Constant/1 -> Add/2
  Add/1 -> Data Type Conversion/1
  Time/1 -> Add/1

== system NCS_Library/Network/Gateway/Gateway1/Ethernet Interface/Subsystem4/Save num release ==
  Time : Inport
  Enable : EnablePort
  Add : Sum
  Constant : Constant  OutDataTypeStr=uint32
  Data Type Conversion : DataTypeConversion  OutDataTypeStr=double
  Display : Display
  Out1 : Outport  InitialOutput=0
  wires:
  Time/1 -> Add/1
  Add/1 -> Data Type Conversion/1
  Constant/1 -> Add/2
  Data Type Conversion/1 -> Display/1, Out1/1

== system NCS_Library/Network/Gateway/Gateway1/Ethernet Interface/User Interface/Subsystem1 ==
  In1 : Inport
  Constant : Constant  Value=0  OutDataTypeStr=uint16
  Constant1 : Constant  Value=0  OutDataTypeStr=uint16
  Mux : Mux  Inputs=3
  Out1 : Outport
  wires:
  In1/1 -> Mux/1
  Mux/1 -> Out1/1
  Constant/1 -> Mux/2
  Constant1/1 -> Mux/3

== system NCS_Library/Network/Gateway/Gateway1/Ethernet Interface/User Interface/Subsystem2 ==
  In1 : Inport
  Constant : Constant  Value=0  OutDataTypeStr=uint16
  Constant1 : Constant  Value=0  OutDataTypeStr=uint16
  Mux : Mux  Inputs=3
  Out1 : Outport
  wires:
  Constant1/1 -> Mux/3
  Constant/1 -> Mux/2
  Mux/1 -> Out1/1
  In1/1 -> Mux/1

== system NCS_Library/Network/Gateway/Gateway1/Ethernet Interface/User Interface/Subsystem3 ==
  In1 : Inport
  Constant : Constant  Value=0  OutDataTypeStr=uint16
  Constant1 : Constant  Value=0  OutDataTypeStr=uint16
  Mux : Mux  Inputs=3
  Out1 : Outport
  wires:
  In1/1 -> Mux/1
  Mux/1 -> Out1/1
  Constant/1 -> Mux/2
  Constant1/1 -> Mux/3

== system NCS_Library/Network/Gateway/Gateway2/CAN Interface/CAN Interface/Re-Transmission Control ==
  IN : Inport
  ReTX : Inport  Port=2
  Reset : Inport  Port=3
  Discard Saved Message upon Success : EntityGate  InputPortMessageModes=m,m  OutputPortMessageModes=m  OperatingMode=Release gate
  Entity Sink : EntityTerminator  InputPortMessageModes=m  NumberEntitiesArrived=on
      settings: OutputPortMap=o0
  Re-Transmission Decision : EntityOutputSwitch  InputPortMessageModes=m  OutputPortMessageModes=m,m  SwitchAttributeName=Attribute1
  Re-transmit Saved Message upon Failure : EntityGate  InputPortMessageModes=m,m  OutputPortMessageModes=m  OperatingMode=Release gate
  OUT : Outport
  #TX : Outport  Port=2
  wires:
  Reset/1 -> Discard Saved Message upon Success/1
  ReTX/1 -> Re-transmit Saved Message upon Failure/1
  Entity Sink/1 -> #TX/1
  Discard Saved Message upon Success/1 -> Entity Sink/1
  Re-Transmission Decision/2 -> Discard Saved Message upon Success/2
  Re-transmit Saved Message upon Failure/1 -> OUT/1
  Re-Transmission Decision/1 -> Re-transmit Saved Message upon Failure/2
  IN/1 -> Re-Transmission Decision/1

== system NCS_Library/Network/Gateway/Gateway2/CAN Interface/CAN Interface/Reception Control/Compute ==
  rx_id : Inport  OutDataTypeStr=double  PortDimensions=1
  loss : Inport  Port=2  OutDataTypeStr=double  PortDimensions=1
  rx_rtr : Inport  Port=3  OutDataTypeStr=double  PortDimensions=1
  rx_data : Inport  Port=4  OutDataTypeStr=double  PortDimensions=1
  tx_id : Inport  Port=5  OutDataTypeStr=double  PortDimensions=1
  tx_rtr : Inport  Port=6  OutDataTypeStr=double  PortDimensions=1
  tx_data : Inport  Port=7  OutDataTypeStr=double  PortDimensions=1
  f : TriggerPort  TriggerType=function-call  VariantControl=Variant
      settings: CopyFcn=Stateflow.SLINSF.SimulinkMan.removeBlockPreDeleteFcn  PreDeleteFcn=Stateflow.SLINSF.SimulinkMan.unsafePredeleteFcn
  Lookup Table : Lookup  InputValues=IDRange  Table=2*ones(1,length(IDRange))-IDSubscription  LUTDesignUseExistingBP=off  LUTDesignAbsError=NaN
  MATLAB Function : MATLAB Function  TreatAsAtomicUnit=on
  Sum : Sum  Inputs=|++
  Status : Outport
  Ack : Outport  Port=2
  wires:
  tx_id/1 -> MATLAB Function/4(ID1)
  rx_rtr/1 -> MATLAB Function/2(RTR0)
  rx_id/1 -> MATLAB Function/1(ID0), Lookup Table/1
  Lookup Table/1 -> Sum/1
  loss/1 -> Sum/2, MATLAB Function/7(Loss)
  rx_data/1 -> MATLAB Function/3(Data0)
  tx_data/1 -> MATLAB Function/6(Data1)
  tx_rtr/1 -> MATLAB Function/5(RTR1)
  Sum/1 -> Status/1
  MATLAB Function/1(ACK) -> Ack/1

== system NCS_Library/Network/Gateway/Gateway2/CAN Interface/CAN Interface/Signal To CAN Message ==
  Data : Inport
  Entity Generator : EntityGenerator  OutputPortMessageModes=m  Period=T_Tx_CAN  GenerateEntityAtSimulationStart=off  GenerateAction=[entity.ID,entity.RTR,entity.Size,entity.f_St,entity.CommDelay,entity.Time, entity.SensorType] = initMessage();  AttributeName=ID|RTR|Size|Data|CommDelay|RndLoss  AttributeInitialValue=1|1|1|1|1|0  EntityType=Bus object  EntityTypeName=CAN_Message  EntityPriority=MsgID
  Set the Attributes of Messages : Subsystem  TreatAsAtomicUnit=on
  MsgOut : Outport
  wires:
  Data/1 -> Set the Attributes of Messages/1(InData)
  Entity Generator/1 -> MsgOut/1

== system NCS_Library/Network/Gateway/Gateway2/CAN Interface/CAN Interface/Simulink Function ==
  controlGate : TriggerPort  TriggerType=function-call  IsSimulinkFunction=on  FunctionName=controlGate  FunctionVisibility=scoped  VariantControl=Variant
  Message Send : MessageSend  OutputPortMessageModes=m
      settings: InputPortMap=u1
  u : ArgIn  DisableCoverage=on  ArgumentName=u
  ctrl : Outport
  wires:
  u/1 -> Message Send/1
  Message Send/1 -> ctrl/1

== system NCS_Library/Network/Gateway/Gateway2/CAN Interface/Entry Control/Enabled Subsystem ==
  Enable : EnablePort  StatesWhenEnabling=reset
  Constant : Constant
  Message Send3 : MessageSend  OutputPortMessageModes=m
      settings: InputPortMap=u1
  Out1 : Outport  OutputWhenDisabled=reset  InitialOutput=1
  wires:
  Message Send3/1 -> Out1/1
  Constant/1 -> Message Send3/1

== system NCS_Library/Network/Gateway/Gateway2/CAN Interface/Gate Control/Save last release time1 ==
  Time : Inport
  Enable : EnablePort
  Add : Sum
  Constant : Constant  OutDataTypeStr=uint32
  Data Type Conversion : DataTypeConversion  OutDataTypeStr=double
  Display : Display
  Out1 : Outport  InitialOutput=0
  wires:
  Time/1 -> Add/1
  Add/1 -> Data Type Conversion/1
  Constant/1 -> Add/2
  Data Type Conversion/1 -> Display/1, Out1/1

== system NCS_Library/Network/Gateway/Gateway2/Ethernet Interface/Subsystem4/Save num release ==
  Time : Inport
  Enable : EnablePort
  Add : Sum
  Constant : Constant  OutDataTypeStr=uint32
  Data Type Conversion : DataTypeConversion  OutDataTypeStr=double
  Display : Display
  Out1 : Outport  InitialOutput=0
  wires:
  Data Type Conversion/1 -> Out1/1, Display/1
  Constant/1 -> Add/2
  Add/1 -> Data Type Conversion/1
  Time/1 -> Add/1

== system NCS_Library/Plant (Train)/freier Wagen/Bremskraft Schienenbremse/WB Bremse pro Wagen/Subsystem/Berechnung W ==
  v : Inport
  Constant : Constant  Value=W_opt
  Constant1 : Constant  Value=v_opt
  Divide : Product  Inputs=*/
  Product : Product
  Scope : Scope
  W : Outport
  wires:
  v/1 -> Divide/1
  Constant1/1 -> Divide/2
  Product/1 -> Scope/1, W/1
  Constant/1 -> Product/1
  Divide/1 -> Product/2

== system NCS_Library/Controller/Logic/Braking Controller/konstante Fahrt/WB Bremse pro Wagen/Subsystem/Berechnung W ==
  v : Inport
  Constant : Constant  Value=W_opt
  Constant1 : Constant  Value=v_opt
  Divide : Product  Inputs=*/
  Product : Product
  Scope : Scope
  W : Outport
  wires:
  Divide/1 -> Product/2
  Constant/1 -> Product/1
  Product/1 -> W/1, Scope/1
  Constant1/1 -> Divide/2
  v/1 -> Divide/1

== system NCS_Library/Network/CAN/Logik/Slow_to_Fast/Measurement/Fast Takt/Simulink Function3 ==
  Gate : TriggerPort  TriggerType=function-call  IsSimulinkFunction=on  FunctionName=Gate  FunctionVisibility=scoped  VariantControl=Variant
  Message Send : MessageSend  OutputPortMessageModes=m
      settings: InputPortMap=u1
  u : ArgIn  DisableCoverage=on  ArgumentName=u
  ctrl : Outport  InitialOutput=0
  wires:
  u/1 -> Message Send/1
  Message Send/1 -> ctrl/1

== system NCS_Library/Network/ETB/OSI Layers/SDTv2/Safety Measures/Sink-Time Supervision/Save last time ==
  Time : Inport
  Enable : EnablePort
  Out1 : Outport  InitialOutput=0
  wires:
  Time/1 -> Out1/1

== system NCS_Library/Network/Gateway/Gateway1/CAN Interface/CAN Interface/Signal To CAN Message/Set the Attributes of Messages ==
  InData : Inport
  initMessage : TriggerPort  TriggerType=function-call  IsSimulinkFunction=on  FunctionName=initMessage  FunctionVisibility=scoped  VariantControl=Variant
  CommDelay : Constant  Value=(49+8*MsgSize)/BUSCapacity  SampleTime=-1
  Constant : Constant  Value=SensorType  OutDataTypeStr=uint8
  Digital Clock : DigitalClock  SampleTime=-1
  ID : Constant  Value=MsgID  SampleTime=-1
  RTR : Constant  Value=0  SampleTime=-1
  Size : Constant  Value=MsgSize  SampleTime=-1
  ID~ : ArgOut  ArgumentName=ID
  RTR~ : ArgOut  Port=2  ArgumentName=RTR
  Size~ : ArgOut  Port=3  ArgumentName=Size
  Data : ArgOut  Port=4  PortDimensions=[3 1]  ArgumentName=Data
  CommDelay~ : ArgOut  Port=5  ArgumentName=CommDelay
  Time : ArgOut  Port=6  ArgumentName=Time
  Type : ArgOut  Port=7  OutDataTypeStr=uint8  ArgumentName=Type
  wires:
  InData/1 -> Data/1
  CommDelay/1 -> CommDelay~/1
  ID/1 -> ID~/1
  RTR/1 -> RTR~/1
  Size/1 -> Size~/1
  Digital Clock/1 -> Time/1
  Constant/1 -> Type/1

== system NCS_Library/Network/Gateway/Gateway2/CAN Interface/CAN Interface/Signal To CAN Message/Set the Attributes of Messages ==
  InData : Inport
  initMessage : TriggerPort  TriggerType=function-call  IsSimulinkFunction=on  FunctionName=initMessage  FunctionVisibility=scoped  VariantControl=Variant
  CommDelay : Constant  Value=(49+8*MsgSize)/BUSCapacity  SampleTime=-1
  Constant : Constant  Value=SensorType  OutDataTypeStr=uint8
  Digital Clock : DigitalClock  SampleTime=-1
  ID : Constant  Value=MsgID  SampleTime=-1
  RTR : Constant  Value=0  SampleTime=-1
  Size : Constant  Value=MsgSize  SampleTime=-1
  ID~ : ArgOut  ArgumentName=ID
  RTR~ : ArgOut  Port=2  ArgumentName=RTR
  Size~ : ArgOut  Port=3  ArgumentName=Size
  Data : ArgOut  Port=4  PortDimensions=[3 1]  ArgumentName=Data
  CommDelay~ : ArgOut  Port=5  ArgumentName=CommDelay
  Time : ArgOut  Port=6  ArgumentName=Time
  Type : ArgOut  Port=7  OutDataTypeStr=uint8  ArgumentName=Type
  wires:
  Constant/1 -> Type/1
  Digital Clock/1 -> Time/1
  Size/1 -> Size~/1
  RTR/1 -> RTR~/1
  ID/1 -> ID~/1
  CommDelay/1 -> CommDelay~/1
  InData/1 -> Data/1

== matlab function NCS_Library/Network/ETB/Ethernet_3-port_switch/Determine Port_N/MATLAB Function ==
  data: Anew output; Destination input; y output; Source input; A input; B input; C input; maxn input
function [Anew, y] = findport(Destination,Source,A,B,C,maxn)

for n=1:1:maxn
    if A(n)==Source
        break
    end
end
saven = n - 1
for n=1:1:saven
    A(n+1)=A(n);
end
A(1) = Source;

n = 1;
while n <= maxn
    if A(n) == Destination
        break
    end
    n = n+1;
end
if n > maxn
    n = 1; 
    while n <= maxn
        if B(n)==Destination
            break
        end
        n = n + 1;
    end
    if n > maxn
        n = 1;
        while n <= maxn
            if C(n) == Destination
                break
            end
            n = n + 1;
        end
        if n > maxn
            y = 3;
        else
            y = 2;
        end
    else
        y = 1;
    end
else
    y = 0;
end
Anew = A;
end

== matlab function NCS_Library/Network/ETB/Ethernet_3-port_switch/Determine Port_L/MATLAB Function ==
  data: Anew output; Destination input; y output; Source input; A input; B input; C input; maxn input
function [Anew, y] = findport(Destination,Source,A,B,C,maxn)

for n=1:1:maxn
    if A(n)==Source
        break
    end
end
saven = n - 1
for n=1:1:saven
    A(n+1)=A(n);
end
A(1) = Source;

n = 1;
while n <= maxn
    if A(n) == Destination
        break
    end
    n = n+1;
end
if n > maxn
    n = 1; 
    while n <= maxn
        if B(n)==Destination
            break
        end
        n = n + 1;
    end
    if n > maxn
        n = 1;
        while n <= maxn
            if C(n) == Destination
                break
            end
            n = n + 1;
        end
        if n > maxn
            y = 3;
        else
            y = 2;
        end
    else
        y = 1;
    end
else
    y = 0;
end
Anew = A;
end

== matlab function NCS_Library/Network/ETB/Ethernet_2-port_Switch/Determine Port_L//R/MATLAB Function1 ==
  data: Anew output; Destination input; y output; Source input; A input; B input; maxn input
function [Anew,y] = findport(Destination,Source,A,B,maxn)

for n=1:1:maxn
    if A(n)==Source
        break
    end
end
saven = n - 1
for n=1:1:saven
    A(n+1)=A(n);
end
A(1) = Source;

n = 1;
while n <= maxn
    if A(n) == Destination
        break
    end
    n = n + 1;
end
if n > maxn
    n = 1;
    while n <= maxn
        if B(n)==Destination
            break
        end
        n = n + 1;
    end
    if n > maxn
            y = 2;
    else
            y = 1;
    end
else
    y = 0;
end
Anew = A;
end

== matlab function NCS_Library/Network/ETB/OSI Layers/MAC Controller/BckOffCntrl/MATLAB Function ==
  data: n_collision input; n_collision output; numColl input; Address input; collision input; MACSource input; route output; MACDestination input; bckoffTime output; numColl output; SlotTime input; SEQ input
function [n_collision,route,bckoffTime,numColl] = handleEntity(n_collision,numColl, Address, collision, MACSource, MACDestination, SlotTime, SEQ)
%% This function handles transmit and receive of entities
% For transmitting it is checked, if there is a collison with a another
% entity. If this is the case the porperties for the retry are set
% For receiving it is checked, if the destination address matches with the
% own address or there is a multicast address
%% generate random numbers with seed equals to MACAddress
rng(uint32(Address(2))+SEQ+uint32(numColl));
k = min((numColl+1),10);
r = uint32( (2^k)*rand(1) );

if Address(2) == MACSource
    %% Handle Transmitting
    if collision == 0
        % ok
        route = uint8(2);
        bckoffTime = 0;
    else
        if numColl < 16
            % retry
            route = uint8(4);
            numColl = uint8(numColl+1);           
            bckoffTime = double(r)*SlotTime;
            
        else
            % fail
            route = uint8(5);
            numColl = uint8(numColl+1);
            bckoffTime = 0;
        end
        
        if collision == 1
            % collision was not counted before
            n_collision = n_collision+1;
        end
    end
    
else
    %% Handle Receiving
    if collision == 0 && ( MACDestination == Address(2) || MACDestination == 200 )
        % ok
        route = uint8(1);
        bckoffTime = 0;
    elseif MACDestination == 99 && Address(2) < 100
        % Multicast to Router
        route = uint8(1);
        bckoffTime = 0;
    else
        % fail
        route = uint8(3);
        bckoffTime = 0;
        if collision == 1
            % collision was not counted before
            n_collision = n_collision+1;
        end
    end
end
end % end function

== matlab function NCS_Library/Network/ETB/OSI Layers/MAC Controller/CSMA//CD Exit/MATLAB Function ==
  data: n input; collision output; collision input
function collision = DetectCollisionExit(n, collision)

if collision
    % packet already collided
    % hence nothing left to do
else
    if n > 1
        % more than one packet in bus
        collision = uint8(1);
    else
        collision = uint8(0);
    end
end
end % end function
